simulink model "Assignment_state_space"  (R2021a)
settings: Solver=VariableStepAuto  StartTime=0.0  StopTime=10.0  RelTol=1e-3
settings Model: Creator=Davie  LastModifiedBy=Davie

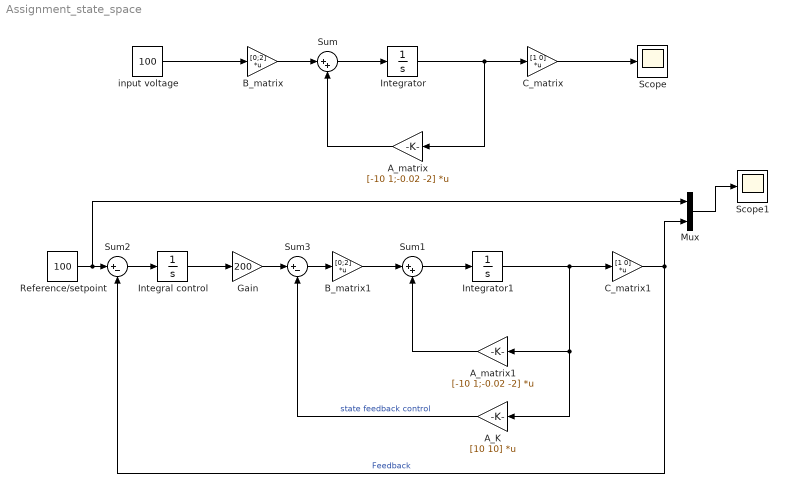
== system Assignment_state_space ==
  A_K : Gain  Gain=[10 10]  Multiplication=Matrix(K*u)
  A_matrix : Gain  Gain=[-10 1;-0.02 -2]  Multiplication=Matrix(K*u)
  A_matrix1 : Gain  Gain=[-10 1;-0.02 -2]  Multiplication=Matrix(K*u)
  B_matrix : Gain  Gain=[0;2]  Multiplication=Matrix(K*u)
  B_matrix1 : Gain  Gain=[0;2]  Multiplication=Matrix(K*u)
  C_matrix : Gain  Gain=[1 0]  Multiplication=Matrix(K*u)
  C_matrix1 : Gain  Gain=[1 0]  Multiplication=Matrix(K*u)
  Gain : Gain  Gain=200
  Integral control : Integrator
  Integrator : Integrator
  Integrator1 : Integrator
  Mux : Mux  Inputs=2
  Reference/setpoint : Constant  Value=100
  Scope : Scope
  Scope1 : Scope
  Sum : Sum  Inputs=|++
  Sum1 : Sum  Inputs=|++
  Sum2 : Sum  Inputs=|+-
  Sum3 : Sum  Inputs=|+-
  input voltage : Constant  Value=100
  wires:
  input voltage/1 -> B_matrix/1
  B_matrix/1 -> Sum/1
  Sum/1 -> Integrator/1
  Integrator/1 -> A_matrix/1, C_matrix/1
  C_matrix/1 -> Scope/1
  A_matrix/1 -> Sum/2
  A_matrix1/1 -> Sum1/2
  Integrator1/1 -> C_matrix1/1, A_K/1, A_matrix1/1
  Sum1/1 -> Integrator1/1
  B_matrix1/1 -> Sum1/1
  Reference/setpoint/1 -> Mux/1, Sum2/1
  Sum2/1 -> Integral control/1
  Sum3/1 -> B_matrix1/1
  A_K/1 -> Sum3/2  "state feedback control"
  Integral control/1 -> Gain/1
  Gain/1 -> Sum3/1
  C_matrix1/1 -> Mux/2, Sum2/2  "Feedback"
  Mux/1 -> Scope1/1
